simulink model "checksimobs"  (R2020b)
settings: Solver=FixedStepAuto  StartTime=0.0  StopTime=inf  FixedStep=0.01  RelTol=1e-3
values from neighbouring files (symbols this model uses):
  cc = cc+1    (= 1)    [Path_planning_run.m]    (also in checkpathplaning.m)
  f_stateg = 0    [Path_planning_run.m]    (also in checkpathplaning.m)
  f_statet = 270    [Path_planning_run.m]    (also in checkpathplaning.m = 180)
  f_statex = 60    [Path_planning_run.m]    (also in checkpathplaning.m = 20)
  f_statey = 64    [Path_planning_run.m]    (also in checkpathplaning.m = 40)
  gammad = [-21 0 21]    [Path_planning_run.m]    (also in checkpathplaning.m)
  i_stateg = 0    [Path_planning_run.m]    (also in checkpathplaning.m)
  i_statet = 180    [Path_planning_run.m]    (also in checkpathplaning.m)
  i_statex = 250    [Path_planning_run.m]    (also in checkpathplaning.m = 200)
  i_statey = 45    [Path_planning_run.m]    (also in checkpathplaning.m = 40)
  IC_theta0 = deg2rad(i_statet)+deg2rad(i_stateg)    [Path_planning_run.m]    (also in checkpathplaning.m)
  IC_theta1 = deg2rad(i_statet)    [Path_planning_run.m]    (also in checkpathplaning.m)
  IC_x0 = x_1f-L_0b*cos(IC_theta0)    [Path_planning_run.m]    (also in checkpathplaning.m)
  IC_x1 = i_statex    (= 250)    [Path_planning_run.m]    (also in checkpathplaning.m = 200)
  IC_y0 = y_1f-L_0b*sin(IC_theta0)    [Path_planning_run.m]    (also in checkpathplaning.m)
  IC_y1 = i_statey    (= 45)    [Path_planning_run.m]    (also in checkpathplaning.m = 40)
  idMO = 1    [checkpathplaning.m]
  L_0b = 0.3    [Path_planning_run.m]    (also in boundingbox_AV.m; check3_dyn.m; checkfinal_dyn.m; checkpathplaning.m)
  L_0f = 3.8    [Path_planning_run.m]    (also in boundingbox_AV.m; check3_dyn.m; checkfinal_dyn.m; checkpathplaning.m)
  L_1f = 8.475    [Path_planning_run.m]    (also in boundingbox_AV.m; check3_dyn.m; checkfinal_dyn.m; checkpathplaning.m)
  lookahead_timeforward = 1.5    [Path_planning_run.m]    (also in checkpathplaning.m = 2)
  lookahead_timereverse = 1.5    [Path_planning_run.m]    (also in checkpathplaning.m)
  lv12_0 = hypot((oh_0b),(w_1/2))    [Path_planning_run.m]    (also in boundingbox_AV.m; check3_dyn.m; checkfinal_dyn.m; checkpathplaning.m)
  lv12_1 = hypot(oh_1b,(w_1/2))    [Path_planning_run.m]    (also in boundingbox_AV.m; check3_dyn.m; checkfinal_dyn.m; checkpathplaning.m)
  lv34_0 = hypot((w_1/2),(L_0f+oh_0f))    [Path_planning_run.m]    (also in boundingbox_AV.m; check3_dyn.m; checkfinal_dyn.m; checkpathplaning.m)
  lv34_1 = hypot((w_1/2),oh_1f)    [Path_planning_run.m]    (also in boundingbox_AV.m; check3_dyn.m; checkfinal_dyn.m; checkpathplaning.m)
  MPFpointx = 160    [checkpathplaning.m]    (also in movingobstacledetection.m)
  MPFpointy = MPSpointy+50    (= 75)    [checkpathplaning.m]    (also in movingobstacledetection.m = 85)
  MPSpointx = 160    [checkpathplaning.m]    (also in movingobstacledetection.m)
  MPSpointy = 25    [checkpathplaning.m]    (also in movingobstacledetection.m)
  obsc = 6    [DPDscenario.m]
  oc = 0    [Path_planning_run.m]    (also in checkpathplaning.m)
  oh_0b = 0.94    [Path_planning_run.m]    (also in boundingbox_AV.m; check3_dyn.m; checkfinal_dyn.m; checkpathplaning.m)
  oh_0f = 1.5    [Path_planning_run.m]    (also in boundingbox_AV.m; check3_dyn.m; checkfinal_dyn.m; checkpathplaning.m)
  oh_1b = 5    [Path_planning_run.m]    (also in boundingbox_AV.m; check3_dyn.m; checkfinal_dyn.m; checkpathplaning.m)
  oh_1f = L_1f+1    (= 9.475)    [Path_planning_run.m]    (also in boundingbox_AV.m; check3_dyn.m; checkfinal_dyn.m; checkpathplaning.m)
  steer_ratioforward = 1    [Path_planning_run.m]    (also in checkpathplaning.m)
  steer_ratioreverse = 1    [Path_planning_run.m]    (also in checkpathplaning.m)
  steer_sensforward = 7.7    [Path_planning_run.m]    (also in checkpathplaning.m = 4)
  steer_sensreverse = 7.2    [Path_planning_run.m]    (also in checkpathplaning.m)
  t_MO = deg2rad(90)    [checkpathplaning.m]    (also in movingobstacledetection.m)
  v_0 = 1    [movingobstacledetection.m]
  w_1 = 2.5    [Path_planning_run.m]    (also in boundingbox_AV.m = 10; check3_dyn.m; checkfinal_dyn.m; checkpathplaning.m)
  xv_lc = [x1_lc x2_lc x3_lc x4_lc]    [Path_planning_run.m]    (also in checkpathplaning.m)
  xv_lg = [x1_lg x2_lg x3_lg x4_lg]    [Path_planning_run.m]    (also in checkpathplaning.m; h_costnewslx.m = ppround_1(xv_lg))
  xv_rv = [61.4 30 30 61.4]    [Path_planning_run.m]    (also in checkpathplaning.m)
  yv_lc = [y1_lc y2_lc y3_lc y4_lc]    [Path_planning_run.m]    (also in checkpathplaning.m)
  yv_lg = [y1_lg y2_lg y3_lg y4_lg]    [Path_planning_run.m]    (also in checkpathplaning.m; h_costnewslx.m = ppround_1(yv_lg))
  yv_rv = [20 20 70 70]    [Path_planning_run.m]    (also in checkpathplaning.m)
undefined symbols (not defined in the file or in its folder): DiscIntNeverNeededParam, g, gfin, gini, obsx, obsy, PP_G, PP_T, PP_X, PP_Y, tfin, timeAV, tini, x, xfin, y, yfin
libraries: vrlib x2, simulink x2
(part 2 of 3)

== matlab function checksimobs/Detection module ==
  data: semi_x input; semi_y input; theta_semi input; gamma input; v_0 input; replanning output; startx_AV output; starty_AV output; starttheta_AV output; startgamma_AV output; startx_MO output; starty_MO output; direction output; MPSpointx parameter; MPSpointy parameter; t_MO parameter; idMO parameter; id input; id output; path input; obsc parameter; obsx parameter; obsy parameter
function [replanning,startx_AV,starty_AV,starttheta_AV,startgamma_AV,startx_MO,starty_MO,direction,id]= fcn(semi_x,semi_y,theta_semi,gamma,v_0,MPSpointx, MPSpointy, t_MO, idMO,id,path,obsc, obsx, obsy)
%_________________________________________________________________________
path1 = rmmissing(path);
pathdir = path1(:,3);
pathx = path1(:,1); % x - values
pathy = path1(:,2); % y - values
paththeta = path1(:,4); % theta-values
pathgamma = path1(:,5); % gamma-values

extx = nan(4000,1);
exty = nan(4000,1);
exttheta = nan(4000,1);
extgamma = nan(4000,1);
path_input = nan(4000,5);
checkarea = nan(1,1);
secondstep = nan(1,1);
replanning = 0;
thirdstep = nan(1,1);
checktime = nan(1,1);
indexcirc = zeros(1,1);
discint_AV = nan(1,1);
startx_AV = nan(1,1);
starty_AV = nan(1,1);
starttheta_AV = nan(1,1);
startgamma_AV = nan(1,1);
startx_MO = nan(1,1);
starty_MO = nan(1,1);
detection = nan(1,1);
%__________________________________________________________________________
xp = semi_x;
yp = semi_y;
thetap = theta_semi;
gammap = gamma;
direction = v_0;
xp_MO = MPSpointx;
yp_MO = MPSpointy;
thetap_MO = t_MO;
movingcollision = collisiondetectionzone(xp,yp,direction,thetap,gammap,xp_MO,yp_MO,thetap_MO);
%__________________________________________________________________________
if movingcollision==1 && id~=idMO
    id = idMO;
    detection = 1;
%__________________________________________________________________________
if detection ==1
   checkdir = pathdir==v_0;
   index = find(checkdir);
   forpathx = pathx(index);
   forpathy = pathy(index);
   forpaththeta = paththeta(index);
   forpathgamma = pathgamma(index);
   x_c1=pchip(linspace(1,length(forpathx),length(forpathx)),forpathx,linspace(1,length(forpathx),length(forpathx)*10)); % interpolate the x- path
   y_c1=pchip(linspace(1,length(forpathy),length(forpathy)),forpathy,linspace(1,length(forpathy),length(forpathy)*10)); % interpolate the y- path
   t_c1=pchip(linspace(1,length(forpaththeta),length(forpaththeta)),forpaththeta,linspace(1,length(forpaththeta),length(forpaththeta)*10)); % interpolate the theta
   g_c1=pchip(linspace(1,length(forpathgamma),length(forpathgamma)),forpathgamma,linspace(1,length(forpathgamma),length(forpathgamma)*10)); % interpolate the gamma
   j = 10;
   d_tot = 0;
   while(d_tot<1.8)
        j=j+1;
        extx=interp1(linspace(1,length(x_c1),length(x_c1)),x_c1,linspace(1,length(x_c1)+(j),length(x_c1)+(j)),'linear','extrap');
        exty=interp1(linspace(1,length(y_c1),length(y_c1)),y_c1,linspace(1,length(y_c1)+(j),length(y_c1)+(j)),'linear','extrap');
        exttheta=interp1(linspace(1,length(t_c1),length(t_c1)),t_c1,linspace(1,length(t_c1)+(j),length(t_c1)+(j)),'linear','extrap');
        extgamma=interp1(linspace(1,length(g_c1),length(g_c1)),g_c1,linspace(1,length(g_c1)+(j),length(g_c1)+(j)),'linear','extrap');
    %     extx=extx';
%     exty=exty';
        d = hypot(diff(extx(length(x_c1):length(extx))),diff(exty(length(y_c1):length(exty))));
        d_tot = sum (d);
    end
    j=length((~isnan(extx)));

% path_input(:,1) = extx;
% path_input(:,2) = exty;
% path_input(:,3) = zeros(length(path_input(:,1)),1);
path_input((1:j),1)= extx(1,(1:j));
path_input((1:j),2) = exty(1,(1:j));% When directon changes simulate 
path_input(:,3) = zeros(1,length(path_input(:,1)));
path_input((1:j),4) = exttheta(1, (1:j));
path_input((1:j),5) = extgamma(1, (1:j));
end
%__________________________________________________________________________
% MPSpointx = MPSpointx; % start point of moving obstacle (x)
% MPSpointy = yp_MO; % start point of moving obstacle (y)
t_MO = deg2rad(t_MO); % orientation of moving obstacle
%__________________________________________________________________________
% assumption that the movement is rectilinear, so arbitray end point is
% selected
MPFpointx = MPSpointx; % final point of moving obstacle (x)
MPFpointy = MPSpointy+50; % final point of moving obstacle (y)

%__________________________________________________________________________
% 
% Way points are decided based on the time dimension. Since the velocity is
% 0.5m/s, for every 1 sec moving obstacle covers half the distance
% compared to an ego (TST) vehicle. In that manner, data points are
% generated
length_MO = sqrt((MPSpointx-MPFpointx)^2+(MPSpointy-MPFpointy)^2);
waypoints = length_MO/0.5;
pathMO_x = linspace(MPSpointx,MPFpointx,waypoints+1);
pathMO_y = linspace(MPSpointy,MPFpointy,waypoints+1);
%__________________________________________________________________________
if detection==1
   pathAV = rmmissing(path_input);
   AV_x = pathAV(:,1);
   AV_y = pathAV(:,2);
   AV_theta = pathAV(:,4);
   AV_gamma = pathAV(:,5);
   a_AV = diff(AV_x); % check diff of AV
   b_AV = diff(AV_y); % check diff of AV
   c_AV = sqrt((a_AV).^2+(b_AV).^2); % calculate distance
   c1_AV = diff(c_AV); % to find any fluctuations
   cc1_AV = round(c1_AV);
   condcc1_AV = any(cc1_AV);
   if condcc1_AV==0
      discint_AV = c_AV(1); % to find discinterval
   end
   disc_AV = 1/discint_AV;
   disc_AV = round(disc_AV);
   indexone_AV = 1:disc_AV:length(AV_x);
   newpathx_AV = AV_x(indexone_AV);
   newpathy_AV = AV_y(indexone_AV);
   newpatht_AV = AV_theta(indexone_AV);
   newpathg_AV = AV_gamma(indexone_AV);
   check_area = checkareafirststep(pathMO_x,pathMO_y,t_MO,AV_x,AV_y,AV_theta,AV_gamma);
   if check_area ==1
      secondstep = 1;
   else
      replanning = 0;
   end
   if secondstep == 1
      [checktime,indexcirc] = checktimesecondstep(AV_x,AV_y,AV_theta,AV_gamma,pathMO_x,pathMO_y,t_MO,newpathx_AV,newpathy_AV,newpatht_AV);
      if checktime ==1
          thirdstep = 1;
      else
          replanning = 0;
      end
   end
   if thirdstep == 1
       indexsuspect = [indexcirc-5 indexcirc-4 indexcirc-3 indexcirc-2 indexcirc-1 indexcirc indexcirc+1 indexcirc+2 indexcirc+3 indexcirc+4 indexcirc+5 indexcirc+6 indexcirc+7 indexcirc+8 indexcirc+9 indexcirc+10 indexcirc+11];
       [startx_AV,starty_AV,starttheta_AV,startgamma_AV,startx_MO,starty_MO] = clashpointfinder(indexsuspect,pathMO_x,pathMO_y,t_MO,newpathx_AV,newpathy_AV,newpatht_AV,newpathg_AV,AV_x,AV_y,AV_theta,AV_gamma,obsc,obsx,obsy);
       replanning = 1;
       direction = v_0;
   end
else
    replanning = 0;
end    
end
y = 1;

== matlab function checksimobs/Subsystem/MATLAB Function1 ==
  data: path input; noteplan input; ms2replan input; repath input; path_input output; checkgoalx output; checkgoaly output; v_0 output; noteplan output
function [path_input,checkgoalx,checkgoaly,v_0,noteplan] = fcn(path, noteplan,ms2replan, repath)

extx = nan(10000,1);
exty = nan(10000,1);
path_input = nan(10000,3);

path1 = rmmissing(path); % remove nan's from path
path2 = path1(:,3); % direction
path3 = path1(:,1); % x - values
path4 = path1(:,2); % y - values

repath = rmmissing(repath);
repath2 = repath(:,3); % direction
repath3 = repath(:,1); % x - values
repath4 = repath(:,2); % y - values

% to find closet values
checkXPP = repath3(end)==path3;
checkyPP = ismember(round(repath4(end)),path4);
[num, indexPP]= min(abs(repath3(end)-path3));
PPend_X = path3(indexPP);

% To have motion primitives in intervals of 21, the below lines are
% performed. In future, the whole script to be changed (in my work, only
% parallel primitives are considered, but it has to be changed with low
% level planner which have to iteratively find an optimal path in complex
% situations)
if indexPP<63
    diffMP = abs(42-indexPP);
else
    diffMP = abs(63-indexPP);
end
intermediate_x = (linspace(repath3(end)+0.01,path3(indexPP+1)-0.01,diffMP))';
intermediate_y = (linspace(repath4(end),path4(indexPP+1),diffMP))';
intermediate_dir  = (linspace(repath2(end),path2(indexPP+1),diffMP))';

intermediate_x1 = (linspace(repath3(end),path3(indexPP),diffMP))';
intermediate_y1 = (linspace(repath4(end),path4(indexPP),diffMP))';
intermediate_dir1  = (linspace(repath2(end),path2(indexPP),diffMP))';
% find final path
if PPend_X<repath3(end)
    finalPATH_X = [repath3;intermediate_x;path3(indexPP+1:length(path3))];
    finalPATH_Y = [repath4;intermediate_y;path4(indexPP+1:length(path4))];
    finalPATH_dir = [repath2;intermediate_dir;path2(indexPP+1:length(path2))];
else
    finalPATH_X = [repath3;intermediate_x1;path3(indexPP:length(path3))];
    finalPATH_Y = [repath4;intermediate_y1;path4(indexPP:length(path4))];
    finalPATH_dir = [repath2;intermediate_dir1;path2(indexPP:length(path2))];
end

forpathx = finalPATH_X;
forpathy = finalPATH_Y;
forpathv = finalPATH_dir;


% MPresolution = 21;
% indexcheck = length(finalPATH_X)/MPresolution; % total number of MP's
% startdis = linspace(1,length(finalPATH_X)-(MPresolution-1),indexcheck);
% enddisc = linspace(21,length(finalPATH_X),indexcheck);
% % anote = startdis(noteplan);
% % enote = enddisc(noteplan);
% anote = startdis(1);
% enote = enddisc(1);
% if ms2replan==1
%     forpathx = finalPATH_X(anote:enote);
%     forpathy = finalPATH_Y(anote:enote);
%     forpathv = finalPATH_dir(anote);
% %     forpathy = finalPATH_Y(startdis(noteplan):enddisc(noteplan));
% %     forpathv = finalPATH_dir(startdis(noteplan));
% else
%     forpathx = finalPATH_X(startdis(noteplan):enddisc(noteplan));
%     forpathy = finalPATH_Y(startdis(noteplan):enddisc(noteplan));
%     forpathv = finalPATH_dir(startdis(noteplan));
% end

if forpathv==1
    v_0 = 1;% velocity
else
    v_0 = -1;
end

x_c1=pchip(linspace(1,length(forpathx),length(forpathx)),forpathx,linspace(1,length(forpathx),length(forpathx)*5)); % interpolate the x- path
y_c1=pchip(linspace(1,length(forpathy),length(forpathy)),forpathy,linspace(1,length(forpathy),length(forpathy)*5)); % interpolate the y- path
checkgoalx = x_c1(end);
checkgoaly = y_c1(end);

j = 10;
d_tot = 0;

while(d_tot<1.8)
    j=j+1;
    extx=interp1(linspace(1,length(x_c1),length(x_c1)),x_c1,linspace(1,length(x_c1)+(j),length(x_c1)+(j)),'linear','extrap');
    exty=interp1(linspace(1,length(y_c1),length(y_c1)),y_c1,linspace(1,length(y_c1)+(j),length(y_c1)+(j)),'linear','extrap');
%     extx=extx';
%     exty=exty';
    d = hypot(diff(extx(length(x_c1):length(extx))),diff(exty(length(y_c1):length(exty))));
    d_tot = sum (d);
end
j=length((~isnan(extx)));

% path_input(:,1) = extx;
% path_input(:,2) = exty;
% path_input(:,3) = zeros(length(path_input(:,1)),1);
path_input((1:j),1)= extx(1,(1:j));
path_input((1:j),2) = exty(1,(1:j));% When directon changes simulate 
path_input(:,3) = zeros(1,length(path_input(:,1)));

noteplan = noteplan; % for next iteration

== matlab function checksimobs/Path extraction/Preparing the path to controller ==
  data: path_input output; path input; checkgoalx output; checkgoaly output; v_0 output; ms2 input; note input; note output
function [path_input,checkgoalx,checkgoaly,v_0,note] = fcn(path,ms2,note)
extx = nan(10000,1);
exty = nan(10000,1);
path_input = nan(10000,3);


% removing NaN from the path extracted
path1 = rmmissing(path); % remove nan's from path
path2 = path1(:,3); % direction
path3 = path1(:,1); % x - values
path4 = path1(:,2); % y - values





% if replan == 1
%     repath = rmmissing(repath);
% repath2 = repath(:,3); % direction
% repath3 = repath(:,1); % x - values
% repath4 = repath(:,2); % y - values
% 
% % to find closet values
% checkXPP = repath3(end)==path3;
% checkyPP = ismember(round(repath4(end)),path4);
% [num, indexPP]= min(abs(repath3(end)-path3));
% PPend_X = path3(indexPP);
% 
% % To have motion primitives in intervals of 21, the below lines are
% % performed. In future, the whole script to be changed (in my work, only
% % parallel primitives are considered, but it has to be changed with low
% % level planner which have to iteratively find an optimal path in complex
% % situations)
% if indexPP<63
%     diffMP = abs(42-indexPP);
% else
%     diffMP = abs(63-indexPP);
% end
% intermediate_x = (linspace(repath3(end)+0.01,path3(indexPP+1)-0.01,diffMP))';
% intermediate_y = (linspace(repath4(end),path4(indexPP+1),diffMP))';
% intermediate_dir  = (linspace(repath2(end),path2(indexPP+1),diffMP))';
% 
% intermediate_x1 = (linspace(repath3(end),path3(indexPP),diffMP))';
% intermediate_y1 = (linspace(repath4(end),path4(indexPP),diffMP))';
% intermediate_dir1  = (linspace(repath2(end),path2(indexPP),diffMP))';
% 
% % find final path
% if PPend_X<repath3(end)
%     finalPATH_X = [repath3;intermediate_x;path3(indexPP+1:length(path3))];
%     finalPATH_Y = [repath4;intermediate_y;path4(indexPP+1:length(path4))];
%     finalPATH_dir = [repath2;intermediate_dir;path2(indexPP+1:length(path2))];
% else
%     finalPATH_X = [repath3;intermediate_x1;path3(indexPP:length(path3))];
%     finalPATH_Y = [repath4;intermediate_y1;path4(indexPP:length(path4))];
%     finalPATH_dir = [repath2;intermediate_dir1;path2(indexPP:length(path2))];
% end
%     finalpath_x  = finalPATH_X;
%     finalpath_y = finalPATH_Y;
%     finalpath_dir = finalPATH_dir;
% else
    finalpath_x = path3;
    finalpath_y = path4;
    finalpath_dir = path2;
% end


MPresolution = 21;
indexcheck = length(path3)/MPresolution; % total number of MP's
% index = 1:1:indexcheck; 
startdis = linspace(1,length(path3)-(MPresolution-1),indexcheck);
% startdis = round(startdis);
enddisc = linspace(21,length(path3),indexcheck);
anote = startdis(note);
enote = enddisc(note);
% enddisc = round(enddisc);
% ass =  note
if ms2==1
%     note = index(1);
    forpathx = finalpath_x(anote:enote);
    forpathy = finalpath_y(startdis(note):enddisc(note));
    forpathv = finalpath_dir(startdis(note));
else
%     note = note+1
    forpathx = finalpath_x(startdis(note):enddisc(note));
    forpathy = finalpath_y(startdis(note):enddisc(note));
    forpathv = finalpath_dir(startdis(note));
%     startdis(1,:) = [];
%     enddisc(1,:) = [];
end
% if ms2==1
% %     note = index(1);
%     forpathx = path3(anote:enote);
%     forpathy = path4(startdis(note):enddisc(note));
%     forpathv = path2(startdis(note));
% else
% %     note = note+1
%     forpathx = path3(startdis(note):enddisc(note));
%     forpathy = path4(startdis(note):enddisc(note));
%     forpathv = path2(startdis(note));
% %     startdis(1,:) = [];
% %     enddisc(1,:) = [];
% end
if forpathv==1
    v_0 = 1;% velocity
else
    v_0 = -1;
end

x_c1=pchip(linspace(1,length(forpathx),length(forpathx)),forpathx,linspace(1,length(forpathx),length(forpathx)*10)); % interpolate the x- path
y_c1=pchip(linspace(1,length(forpathy),length(forpathy)),forpathy,linspace(1,length(forpathy),length(forpathy)*10)); % interpolate the y- path
checkgoalx = x_c1(end);
checkgoaly = y_c1(end);
% x_c11 = x_c1';
% y_c11 = y_c1';
j = 10;
d_tot = 0;

while(d_tot<1.8)
    j=j+1;
    extx=interp1(linspace(1,length(x_c1),length(x_c1)),x_c1,linspace(1,length(x_c1)+(j),length(x_c1)+(j)),'linear','extrap');
    exty=interp1(linspace(1,length(y_c1),length(y_c1)),y_c1,linspace(1,length(y_c1)+(j),length(y_c1)+(j)),'linear','extrap');
%     extx=extx';
%     exty=exty';
    d = hypot(diff(extx(length(x_c1):length(extx))),diff(exty(length(y_c1):length(exty))));
    d_tot = sum (d);
end
j=length((~isnan(extx)));

% path_input(:,1) = extx;
% path_input(:,2) = exty;
% path_input(:,3) = zeros(length(path_input(:,1)),1);
path_input((1:j),1)= extx(1,(1:j));
  path_input((1:j),2) = exty(1,(1:j));% When directon changes simulate 
         path_input(:,3) = zeros(1,length(path_input(:,1)));
         note = note; % for next iteration

== matlab function checksimobs/STop simulation1/Stop simulation2 ==
  data: checkgoalx input; y1 output; checkgoaly input; semi_x input; semi_y input; ms3 output; ms2 output; xv_lc parameter; yv_lc parameter; note output; note input
function [y1,ms3,ms2,note] = fcn(checkgoalx,checkgoaly,semi_x,semi_y,xv_lc, yv_lc,note)
ms3 =0;     % Disable Path extraction subsystem
ms2 = 1;    % Currently, keeping first index constant
% note = 1;
coder.extrinsic('InPolygon');
% areacond = false(1,1);
in = InPolygon(checkgoalx,checkgoaly,xv_lc,yv_lc); % check whether cur is in the zone
% areacond = any(in);
% if ~in && abs(checkgoalx-semi_x)<0.1 && abs(checkgoaly-semi_y)<0.1
Acheck = abs(checkgoalx-semi_x);
Bcheck = abs(checkgoaly-semi_y);
if ~in && Acheck<0.1 && Bcheck<0.1
    ms3 = 1; % activate path extraction subsystem for changing the path
    ms2 = 0; % activate change in path - path extraction subsystem
    y1 = 0;  % disable to stop simulation 
    note = note+1; % to update the next index to chose
%     path_input = 0;    
elseif in && Acheck<0.1 && Bcheck<0.1
    y1 = 1; % to stop the simulation
else
    ms3 = 0; % de-activate path extraction subsystem
    y1 = 0;  % disable to stop simulation
end

== matlab function checksimobs/Controller/Forward controller/Embedded MATLAB Function ==
  settings: updateMethod=DISCRETE
  data: path_input input; point input; dist output; npoints input; pos output; idx2 output; idx1 input; alpha output; b_dist output; worldchanged input
function [dist,pos,idx2,alpha,b_dist] = dist2path(path_input,point,npoints,idx1,worldchanged)

persistent a b c idx mdist dist_sgn
path = rmmissing(path_input);
path = path';
asas = size(path);
a=[0 0 0]';
b=[0 0 0]';
c=[0 0 0]';
pos=[0 0 0]';
b_dist=[0 0 0]';
mdist=[0];
idx=0;
if worldchanged==0
idx=idx1;
end
% idx=idx1;
alpha=[0];

%Determination of idx_min and idx_max : plage de [idx-npoints,idx+npoints]
%npoints=10
if idx<0
    idx_min=1;
    idx_max=length(path);
else
    idx_min=max(1,idx-npoints);
    idx_max=min(length(path),idx+npoints);
end
% sds = idx_min
% asd = idx_max
% idx_min_dist=0;
min_dist=1e8;
ass = point;
%Determination of the shortest path to the closest reference point
for i=idx_min:idx_max
    mdist=norm(path(:,i) - point);  % Distance viewpoint to reference path for all reference points
    if mdist<min_dist               % If distance is smaller than previous distance
        idx=i;                      % Shortest path is reference point i            
        min_dist=mdist;         	% Shortest distance is updated 
        pos=path(:,i);          	% Reference point on reference path is updated.
    end
end

%Indice   Keeping reference point inside the reference path
idx=max(idx,2);
idx=min(idx,length(path)-1);


for i=idx-1:idx      
    a=path(:,i+1)-path(:,i);    %[dx dy dz] of distance between minimal ref point and previous point
    b=point-path(:,i);          % distance between reaction point and reference point
    
    b_dist=b;
    alpha=dot(a,b)/dot(a,a);    %product vectors a,b /  product vectors a,a -> rapport distance a et projection de b sur a
    dist=norm(b-alpha*a);       %distance avec la trajectoire droite entre les deux points
    
    if alpha > 0 && alpha < 1 && dist < min_dist %Le vehicule est avant le point vise  
        min_dist=dist;  %Distance mini
        pos=path(:,i)+alpha*a;  %point reellement vise
        idx=i;              
        c=cross(a,b);       %produit vectoriel  
        dist_sgn=sign(c(3));        %signe du produit vectoriel au niveau de Z
    end
end

a= path(:,idx+1) - path(:,idx);
b= point - pos;
c= cross(a,b);
dist_sgn=sign(c(3));

dist= min_dist*dist_sgn;
idx2=idx;

== matlab function checksimobs/Controller/Forward controller/Subsystem/MATLAB Function ==
  settings: updateMethod=DISCRETE
  data: path_input input; dist output; point input; npoints input; idx1 input; pos output; idx2 output; alpha output; b_dist output
function [dist,pos,idx2,alpha,b_dist] = dist2path(path_input,point,npoints,idx1)
%#eml
path = rmmissing(path_input);
path = path';
persistent a b c idx mdist dist_sgn

a=[0 0 0]';
b=[0 0 0]';
c=[0 0 0]';
pos=[0 0 0]';
b_dist=[0 0 0]';
mdist=[0];
idx=0;

idx=idx1;
alpha=[0];

%Determination of idx_min and idx_max : plage de [idx-npoints,idx+npoints]
%npoints=10
if idx<0
    idx_min=1;
    idx_max=length(path);
else
    idx_min=max(1,idx-npoints);
    idx_max=min(length(path),idx+npoints);
end

% idx_min_dist=0;
min_dist=1e8;

%Determination of the shortest path to the closest reference point
for i=idx_min:idx_max
    mdist=norm(path(:,i) - point);  % Distance viewpoint to reference path for all reference points
    if mdist<min_dist               % If distance is smaller than previous distance
        idx=i;                      % Shortest path is reference point i            
        min_dist=mdist;         	% Shortest distance is updated 
        pos=path(:,i);          	% Reference point on reference path is updated.
    end
end

%Indice   Keeping reference point inside the reference path
idx=max(idx,2);
idx=min(idx,length(path)-1);


for i=idx-1:idx      
    a=path(:,i+1)-path(:,i);    %[dx dy dz] of distance between minimal ref point and previous point
    b=point-path(:,i);          % distance between reaction point and reference point
    
    b_dist=b;
    alpha=dot(a,b)/dot(a,a);    %product vectors a,b /  product vectors a,a -> rapport distance a et projection de b sur a
    dist=norm(b-alpha*a);       %distance avec la trajectoire droite entre les deux points
    
    if alpha > 0 && alpha < 1 && dist < min_dist %Le vehicule est avant le point vise  
        min_dist=dist;  %Distance mini
        pos=path(:,i)+alpha*a;  %point reellement vise
        idx=i;              
        c=cross(a,b);       %produit vectoriel  
        dist_sgn=sign(c(3));        %signe du produit vectoriel au niveau de Z
    end
end

a= path(:,idx+1) - path(:,idx);
b= point - pos;
c= cross(a,b);
dist_sgn=sign(c(3));

dist= min_dist*dist_sgn;
idx2=idx;

== matlab function checksimobs/Inverse kinematics model/IK_function ==
  data: x_1 input; y_1 input; theta_0 input; theta_1 input; x_1_dot output; L_0b parameter; L_1f parameter; gamma_1 input; y_1_dot output; theta_0_dot output; theta_1_dot output; v_1 input; x_0f output; y_0f output; x_0 output; y_0 output; x_1f output; y_1f output; v_0 output; delta_C input; L_0f parameter; delta_I2K output
% The vehicle is described in global coordinates for which ISO system is used.
% Yaw rates can be derived from applying non-holonomic consraint (no lateral
% slip) on each axle.

function [x_1_dot,y_1_dot,theta_0_dot,theta_1_dot,x_0f,y_0f,x_0,y_0,x_1f,y_1f,...
         v_0,delta_I2K] = vehicle(x_1,y_1,theta_0,theta_1,L_0b,L_1f,gamma_1,v_1,delta_C,L_0f)
     
%_______________________ position _________________________________________
%king-pin

        x_1f = x_1+L_1f*cos(theta_1);
        y_1f = y_1+L_1f*sin(theta_1);

 
% drive axle

        x_0 = x_1f-L_0b*cos(theta_0);
        y_0 = y_1f-L_0b*sin(theta_0);

% steer axle

        x_0f = x_0+L_0f*cos(theta_0);
        y_0f = y_0+L_0f*sin(theta_0);
                       
% yaw rate        
                                      
        theta_1_dot = abs(v_1)*tan(delta_C)/L_1f;                           % semitrailer
        theta_0_dot = sign(v_1)*sign(L_0b)*(-(v_1/L_0b)*sin(gamma_1)+...
                    (L_1f/L_0b)*(theta_1_dot)*cos(gamma_1));                % tractor 
                      
% semitrailer longitudinal velocity in its own local body coordinate system

        v_0 = v_1*cos(gamma_1) + L_1f*(theta_1_dot)*sin(gamma_1); 
        
        delta_I2K = atan(L_0f*theta_0_dot/v_0);
                    
        
%_________________________next iteration___________________________________
        
        x_1_dot = v_1 * cos(theta_1);                                       % tractor drive axle velocity in global x-direction
        y_1_dot = v_1 * sin(theta_1);                                       % tractor drive axle velocity in global y-direction

== matlab function checksimobs/Kinematic model/KM function ==
  data: x_0 input; y_0 input; theta_0 input; theta_1 input; x_0_dot output; L_0b parameter; L_1f parameter; y_0_dot output; theta_0_dot output; theta_1_dot output; v_0 input; x_0f output; y_0f output; x_1f output; y_1f output; x_1 output; y_1 output; gamma_1 output; v_1 output; delta input; L_0f parameter
% The vehicle is described in global coordinates for which ISO system is used.
% Yaw rates can be derived from applying non-holonomic consraint (no lateral
% slip) on each axle.

function [x_0_dot,y_0_dot,theta_0_dot,theta_1_dot,x_0f,y_0f,x_1f,y_1f,x_1,y_1,gamma_1,...
         v_1] = vehicle(x_0,y_0,theta_0,theta_1,L_0b,L_1f,v_0,delta,L_0f)
     
%_______________________ position _________________________________________
% steer axle

        x_0f = x_0+L_0f*cos(theta_0);
        y_0f = y_0+L_0f*sin(theta_0);
        
%king-pin

        x_1f = x_0+L_0b*cos(theta_0);
        y_1f = y_0+L_0b*sin(theta_0);
 
% semitrailer axle

        x_1 = x_1f-L_1f*cos(theta_1);
        y_1 = y_1f-L_1f*sin(theta_1);
        
% articulation angle
        
        gamma_1 = (theta_0-theta_1);                                        % articulation angle
        
% yaw rate        
        
        theta_0_dot = (v_0/L_0f) * tan(delta);                              % tractor 
        theta_1_dot = (v_0/L_1f)*sin(gamma_1) + (L_0b/L_1f)*...
                        (theta_0_dot)*cos(gamma_1);                         % semitrailer                            
                    
                    
% semitrailer longitudinal velocity in its own local body coordinate system

        v_1 = v_0*cos(gamma_1) - L_0b*(theta_0_dot)*sin(gamma_1);  
                    
        
%_________________________next iteration____________________________________
        
        x_0_dot = v_0 * cos(theta_0);                                          % tractor drive axle velocity in global x-direction
        y_0_dot = v_0 * sin(theta_0);                                          % tractor drive axle velocity in global y-direction

== matlab function checksimobs/Controller/Reverse controller/Embedded MATLAB Function ==
  settings: updateMethod=DISCRETE
  data: path_input input; point input; dist output; npoints input; pos output; idx2 output; idx1 input; alpha output; b_dist output; worldchanged input
function [dist,pos,idx2,alpha,b_dist] = dist2path(path_input,point,npoints,idx1,worldchanged)
%#eml
path = rmmissing(path_input);
path = path';
persistent a b c idx mdist dist_sgn

a=[0 0 0]';
b=[0 0 0]';
c=[0 0 0]';
pos=[0 0 0]';
b_dist=[0 0 0]';
mdist=[0];
% idx=0;
% 
% idx=idx1;
if worldchanged==1
idx=0;
else
    idx=idx1;
end
alpha=[0];

%Determination of idx_min and idx_max : plage de [idx-npoints,idx+npoints]
%npoints=10
if idx<0
    idx_min=1;
    idx_max=length(path);
else
    idx_min=max(1,idx-npoints);
    idx_max=min(length(path),idx+npoints);
end

% idx_min_dist=0;
min_dist=1e8;

%Determination of the shortest path to the closest reference point
for i=idx_min:idx_max
    mdist=norm(path(:,i) - point);  % Distance viewpoint to reference path for all reference points
    if mdist<min_dist               % If distance is smaller than previous distance
        idx=i;                      % Shortest path is reference point i            
        min_dist=mdist;         	% Shortest distance is updated 
        pos=path(:,i);          	% Reference point on reference path is updated.
    end
end

%Indice   Keeping reference point inside the reference path
idx=max(idx,2);
idx=min(idx,length(path)-1);


for i=idx-1:idx      
    a=path(:,i+1)-path(:,i);    %[dx dy dz] of distance between minimal ref point and previous point
    b=point-path(:,i);          % distance between reaction point and reference point
    
    b_dist=b;
    alpha=dot(a,b)/dot(a,a);    %product vectors a,b /  product vectors a,a -> rapport distance a et projection de b sur a
    dist=norm(b-alpha*a);       %distance avec la trajectoire droite entre les deux points
    
    if alpha > 0 && alpha < 1 && dist < min_dist %Le vehicule est avant le point vise  
        min_dist=dist;  %Distance mini
        pos=path(:,i)+alpha*a;  %point reellement vise
        idx=i;              
        c=cross(a,b);       %produit vectoriel  
        dist_sgn=sign(c(3));        %signe du produit vectoriel au niveau de Z
    end
end

a= path(:,idx+1) - path(:,idx);
b= point - pos;
c= cross(a,b);
dist_sgn=sign(c(3));

dist= min_dist*dist_sgn;
idx2=idx;

== matlab function checksimobs/Controller/Reverse controller/Subsystem/MATLAB Function ==
  settings: updateMethod=DISCRETE
  data: path_input input; dist output; point input; npoints input; idx1 input; pos output; idx2 output; alpha output; b_dist output
function [dist,pos,idx2,alpha,b_dist] = dist2path(path_input,point,npoints,idx1)
%#eml
path = rmmissing(path_input);
path = path';
persistent a b c idx mdist dist_sgn

a=[0 0 0]';
b=[0 0 0]';
c=[0 0 0]';
pos=[0 0 0]';
b_dist=[0 0 0]';
mdist=[0];
idx=0;

idx=idx1;
alpha=[0];

%Determination of idx_min and idx_max : plage de [idx-npoints,idx+npoints]
%npoints=10
if idx<0
    idx_min=1;
    idx_max=length(path);
else
    idx_min=max(1,idx-npoints);
    idx_max=min(length(path),idx+npoints);
end

% idx_min_dist=0;
min_dist=1e8;

%Determination of the shortest path to the closest reference point
for i=idx_min:idx_max
    mdist=norm(path(:,i) - point);  % Distance viewpoint to reference path for all reference points
    if mdist<min_dist               % If distance is smaller than previous distance
        idx=i;                      % Shortest path is reference point i            
        min_dist=mdist;         	% Shortest distance is updated 
        pos=path(:,i);          	% Reference point on reference path is updated.
    end
end

%Indice   Keeping reference point inside the reference path
idx=max(idx,2);
idx=min(idx,length(path)-1);


for i=idx-1:idx      
    a=path(:,i+1)-path(:,i);    %[dx dy dz] of distance between minimal ref point and previous point
    b=point-path(:,i);          % distance between reaction point and reference point
    
    b_dist=b;
    alpha=dot(a,b)/dot(a,a);    %product vectors a,b /  product vectors a,a -> rapport distance a et projection de b sur a
    dist=norm(b-alpha*a);       %distance avec la trajectoire droite entre les deux points
    
    if alpha > 0 && alpha < 1 && dist < min_dist %Le vehicule est avant le point vise  
        min_dist=dist;  %Distance mini
        pos=path(:,i)+alpha*a;  %point reellement vise
        idx=i;              
        c=cross(a,b);       %produit vectoriel  
        dist_sgn=sign(c(3));        %signe du produit vectoriel au niveau de Z
    end
end

a= path(:,idx+1) - path(:,idx);
b= point - pos;
c= cross(a,b);
dist_sgn=sign(c(3));

dist= min_dist*dist_sgn;
idx2=idx;

== matlab function checksimobs/Stop simulation1 ==
  data: checkgoalxplan input; y1 output; checkgoalyplan input; semi_x input; semi_y input; ms3replan output; ms2replan output; xv_lc parameter; yv_lc parameter; noteplan output; noteplan input
function [y1,ms3replan,ms2replan,noteplan] = fcn(checkgoalxplan,checkgoalyplan,semi_x,semi_y,xv_lc, yv_lc,noteplan)
ms3replan =0;     % Disable Path extraction subsystem
ms2replan = 1;    % Currently, keeping first index constant

coder.extrinsic('InPolygon');
% areacond = false(1,1);
in = InPolygon(checkgoalxplan,checkgoalyplan,xv_lc,yv_lc); % check whether cur is in the zone
% areacond = any(in);
% if ~in && abs(checkgoalx-semi_x)<0.1 && abs(checkgoaly-semi_y)<0.1
Acheck = abs(checkgoalxplan-semi_x);
Bcheck = abs(checkgoalyplan-semi_y);
% sads = semi_x;
% asdas = semi_y;
% asdsa = checkgoalxplan;
% asddasdas = checkgoalyplan;
if ~in && Acheck<0.1 && Bcheck<0.1
    ms3replan = 1; % activate path extraction subsystem for changing the path
    ms2replan = 0; % activate change in path - path extraction subsystem
    y1 = 0;  % disable to stop simulation 
    noteplan = noteplan+1; % to update the next index to chose
%     path_input = 0;    
elseif in && Acheck<0.1 && Bcheck<0.1
    y1 = 1; % to stop the simulation
else
    ms3replan = 0; % de-activate path extraction subsystem
    y1 = 0;  % disable to stop simulation
%     noteplan = noteplan;
end

== matlab function checksimobs/Obstacle check module/MATLAB Function2 ==
  data: AVx input; AVy input; AVtheta input; AVgamma input; MOx input; MOy input; repath output; MPFpointx parameter; MPFpointy parameter; PP_G parameter; PP_T parameter; PP_X parameter; PP_Y parameter; t_MO parameter; obsc parameter; obsx parameter; obsy parameter; direction input; checkgoalx output; checkgoaly output; y output
function [repath,checkgoalx,checkgoaly,y]= fcn(AVx,AVy,AVtheta,AVgamma,MOx,MOy,MPFpointx, MPFpointy, PP_G, PP_T, PP_X, PP_Y, t_MO, obsc, obsx, obsy, direction)
% a = AVx
% b = AVy
% c = AVtheta
% d = AVgamma
% e = MOx
% f = MOy

checkfin = nan(1,1);
indexfree = nan(1,1);

length_MO1 = sqrt((MOx-MPFpointx)^2+(MOy-MPFpointy)^2);
waypoints1 = length_MO1/0.5;
pathMO_x1 = linspace(MOx,MPFpointx,waypoints1+1);
pathMO_y1 = linspace(MOy,MPFpointy,waypoints1+1);

PPfinaltini = rad2deg(PP_T(1,:));
startthetaAV = rad2deg(AVtheta);
checkPP = startthetaAV ==PPfinaltini;
indexPP = find(checkPP);
% for my convienence splitting the array and then combining it
A_PP = indexPP(1:10);
B_PP = indexPP(11:20);
C_PP = [A_PP(1) B_PP(1) A_PP(2) B_PP(2) A_PP(3) B_PP(3) A_PP(4) B_PP(4) A_PP(5) B_PP(5) A_PP(6) B_PP(6) A_PP(7) B_PP(7) A_PP(8) B_PP(8) A_PP(9) B_PP(9) A_PP(10) B_PP(10)];

for k = 1:length(C_PP)
    xp_clash = AVx+PP_X(:,C_PP(k));
    yp_clash = AVy+PP_Y(:,C_PP(k));
    thetap_clash = PP_T(:,C_PP(k));
    gammap_clash = PP_G(:,C_PP(k));
    for j = 1:length(xp_clash)
        xp = xp_clash(j);
        yp = yp_clash(j);
        thetap = thetap_clash(j);
        gammap = gammap_clash(j);
        xp_MO = pathMO_x1(j);
        yp_MO = pathMO_y1(j);
        thetap_MO = t_MO;
        checkfin = checkfinal_dyn(xp,yp,thetap,gammap,xp_MO,yp_MO,thetap_MO,obsc,obsx,obsy);
        if checkfin==1
           check_k = 1; % intersect
            break;
        else
            check_k = 0; % do not intersect
        end
    end
    if check_k ==0
        indexfree = k;
        break;
    end
end

% Finding new path
finalPATH_XPP = AVx+PP_X(:,C_PP(indexfree+2));
finalPATH_YPP = AVy+PP_Y(:,C_PP(indexfree+2));
finalPATH_THETAPP = PP_T(:,C_PP(indexfree+2));
finalPATH_GAMMAPP = PP_G(:,C_PP(indexfree+2));
finalPATH_direction = direction+zeros(size(finalPATH_XPP));

repath = nan(63,5);
k = 1; 
% for m = i:-1:1
    for j = 1:63
        repath(k,1) = finalPATH_XPP(j);
        repath(k,2) = finalPATH_YPP(j);
        repath(k,3) = finalPATH_direction(j);
        repath(k,4) = finalPATH_THETAPP(j);
        repath(k,5) = finalPATH_GAMMAPP(j);
        k = k+1;
    end
% end
checkgoalx = finalPATH_XPP(1);
checkgoaly = finalPATH_YPP(1);
y = 0;

% y = 1;

== matlab function checksimobs/MATLAB Function ==
  data: stopcheckgoalx input; dynrepath output; stopcheckgoaly input; semi_x input; semi_y input
function dynrepath = fcn(stopcheckgoalx,stopcheckgoaly,semi_x,semi_y)

Acheckreplan = abs(stopcheckgoalx-semi_x);
Bcheckreplan = abs(stopcheckgoaly-semi_y);
% && actfirstsim~=actfirst
if Acheckreplan<0.1 && Bcheckreplan<0.1 
   dynrepath = 1; % to stop the simulation
%     note_replan = note_replan+1; % to update the next index to chose
%    note_replan = note_replan;
else
    dynrepath = 0;
end
% noteplan = 1;

== matlab function checksimobs/Path planner/MATLAB Function3 ==
  data: path input; f_statex parameter; f_statey parameter; ms output; f_statet parameter; ms1 output
function [ms,ms1] = fcn(path, f_statex, f_statey, f_statet)
coder.extrinsic('InPolygon');
path1 = rmmissing(path);
a = path1(end,1);
b = path1(end,2);
lz= 5; % IN zone
wz= 1.5;
dt1= f_statet + atand(wz/lz);
dt2= f_statet - atand(wz/lz);
dl= hypot(wz/2,lz/2);
x1=  f_statex + dl*cosd(dt1);
y1=  f_statey + dl*sind(dt1);
x2=  f_statex + dl*cosd(dt2);
y2=  f_statey + dl*sind(dt2);
x3=  f_statex + dl*cosd(dt1+180);
y3=  f_statey + dl*sind(dt1+180);
x4=  f_statex + dl*cosd(dt2+180);
y4=  f_statey + dl*sind(dt2+180);
xv = [x1 x2 x3 x4];
yv = [y1 y2 y3 y4];
in = InPolygon(a,b,xv,yv); % check whether cur is in the zone
if in
    ms = 0;
    ms1 = 1
else
    ms = 1;
    ms1 = 0;
end
